simulink model "simTraj"  (R2016a)
settings: Solver=VariableStepAuto  StartTime=0.0  StopTime=10.0  RelTol=1e-3
libraries: simulink x1
settings Model: Creator=tim  LastModifiedBy=tim

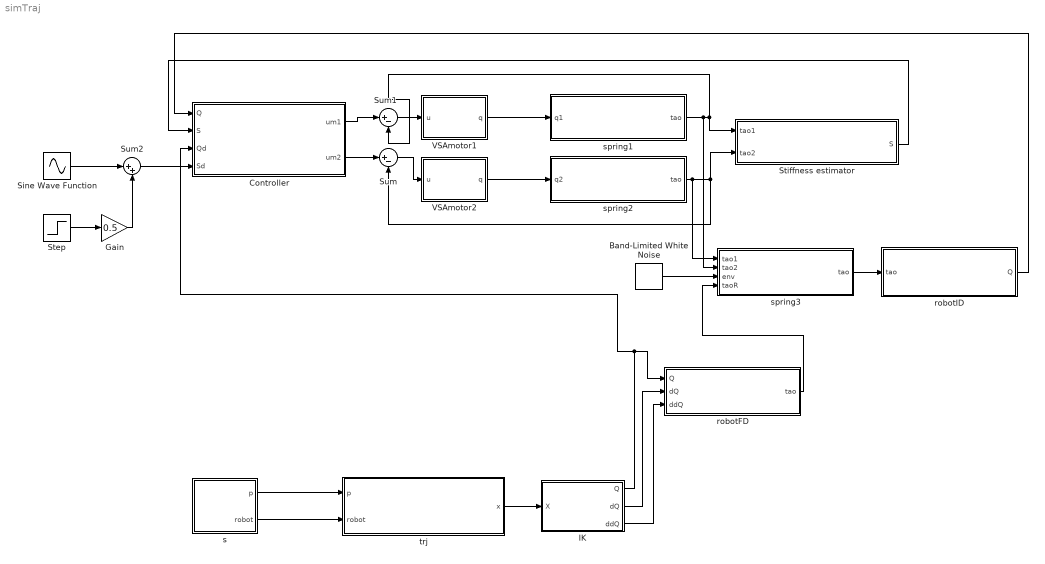
== system simTraj ==
  Band-Limited White Noise : simulink/Sources/Band-Limited White Noise  Cov=[0.1]  Ts=0.1  seed=[23341]
  Controller : MATLAB Function  TreatAsAtomicUnit=on
  Gain : Gain  Gain=0.5
  IK : MATLAB Function  TreatAsAtomicUnit=on
  Sine Wave Function : Sin  TimeSource=Use external signal  Amplitude=0.3  SampleTime=0
  Step : Step  SampleTime=0
  Stiffness estimator : MATLAB Function  TreatAsAtomicUnit=on
  Sum : Sum  Inputs=|+-
  Sum1 : Sum  Inputs=|+-
  Sum2 : Sum  Inputs=|++
  VSAmotor1 : MATLAB Function  TreatAsAtomicUnit=on
  VSAmotor2 : MATLAB Function  TreatAsAtomicUnit=on
  robotFD : MATLAB Function  TreatAsAtomicUnit=on
  robotID : MATLAB Function  TreatAsAtomicUnit=on
  s : MATLAB Function  TreatAsAtomicUnit=on
  spring1 : MATLAB Function  TreatAsAtomicUnit=on
  spring2 : MATLAB Function  TreatAsAtomicUnit=on
  spring3 : MATLAB Function  TreatAsAtomicUnit=on
  trj : MATLAB Function  TreatAsAtomicUnit=on
  wires:
  s/1(p) -> trj/1(p)
  trj/1(x) -> IK/1(X)
  IK/2(dQ) -> robotFD/2(dQ)
  IK/3(ddQ) -> robotFD/3(ddQ)
  IK/1(Q) -> robotFD/1(Q), Controller/3(Qd)
  Sine Wave Function/1 -> Sum2/1
  s/2(robot) -> trj/2(robot)
  Controller/1(um1) -> Sum1/1
  Controller/2(um2) -> Sum/1
  VSAmotor1/1(q) -> spring1/1(q1)
  VSAmotor2/1(q) -> spring2/1(q2)
  Stiffness estimator/1(S) -> Controller/2(S)
  Sum/1 -> VSAmotor2/1(u)
  spring1/1(tao) -> spring3/2(tao2), Stiffness estimator/1(tao1), Sum1/2
  spring2/1(tao) -> spring3/1(tao1), Stiffness estimator/2(tao2), Sum/2
  Sum1/1 -> VSAmotor1/1(u)
  Band-Limited White Noise/1 -> spring3/3(env)
  spring3/1(tao) -> robotID/1(tao)
  robotID/1(Q) -> Controller/1(Q)
  robotFD/1(tao) -> spring3/4(taoR)
  Sum2/1 -> Controller/4(Sd)
  Step/1 -> Gain/1
  Gain/1 -> Sum2/2

== matlab function simTraj/Controller ==
  data: Q input; um1 output; S input; Qd input; Sd input; um2 output
function [um1,um2] = dec_vsa_controller(Q,S,Qd,Sd)

    [um1 um2] = decenterController(Q,S,Qd,Sd);

end

== matlab function simTraj/trj ==
  data: p input; x output; robot input
function x = trajectory_planning(p,robot)
    x = trajectory(p,robot);
end

== matlab function simTraj/IK ==
  data: X input; Q output; dQ output; ddQ output
function [Q,dQ,ddQ] = Inverse(X)
    Q = IK(X);
    dQ = [Q(2:end,:);0 0] - [0 0;Q(1:end-1,:)];
    ddQ = [dQ(2:end,:);0 0] - [0 0;dQ(1:end-1,:)];
end

== matlab function simTraj/s ==
  data: p output; robot output
function [p,robot] = setup()
    %translation vector from frame to frame
robot.L(1,:) = [5 0]; 
robot.L(2,:) = [4 0];

%translation to the COM of the link from the end 
robot.COM(1,:) = [-3 0 0];
robot.COM(2,:) = [-2.2 0 0];

%restrictions for the linear and angular speed
robot.VCartEE = 2;
% robot.VJoint(1) = 1;
% robot.VJoint(2) = 1;
% robot.VJoint(3) = 1;
%here we focused only on the Cartesian velocity constrains

robot.M(1) = 3;
robot.M(2) = 2;
robot.I(1) = 2.5;
robot.I(2) = 1.5;

%200 Hz
robot.Freq = 200;

%trajectory of the robot will be closed in this triangle
p = [4,4;
    5,6;
    2,3;
    4,4];
%plotting trajectory

end

== matlab function simTraj/VSAmotor1 ==
  data: u input; q output
function q = motor1(u)
%#codegen

q = u;

== matlab function simTraj/VSAmotor2 ==
  data: u input; q output
function q = motor2(u)
%#codegen

q = u;

== matlab function simTraj/Stiffness estimator ==
  data: tao1 input; S output; tao2 input
function S = springs_stiffness_actuators(tao1,tao2)
%#codegen

S = tao1+tao2;

== matlab function simTraj/spring1 ==
  data: q1 input; tao output
function tao = spring1(q1)
%#codegen

tao=q1;

== matlab function simTraj/spring2 ==
  data: q2 input; tao output
function tao = spring2(q2)
%#codegen

tao=q2;

== matlab function simTraj/spring3 ==
  data: tao1 input; tao2 input; tao output; env input; taoR input
function tao = jTorque(tao1,tao2,env,taoR)
%#codegen

tao=tao1+tao2+env+taoR;

== matlab function simTraj/robotID ==
  data: tao input; Q output
function Q = robot(tao)
%#codegen

Q = ID(tao);

== matlab function simTraj/robotFD ==
  data: tao output; Q input; dQ input; ddQ input
function tao = robot(Q,dQ,ddQ)
%robot forward Dynamics

tao = FD(Q,dQ,ddQ);
